simulink library "module_switch"  (R2013b)
settings: Solver=ode45  StartTime=0.0  StopTime=10.0  RelTol=1e-3
values from neighbouring files (symbols this model uses):
  D = (Vref - Vs) / Vref    (= 0.6)    [array_init.m]
  modes = 4    [array_init.m]
  T = 4e-6    (= 4e-06)    [array_init.m]
  Tstartup = 3e-3    (= 0.003)    [array_init.m]
libraries: fl_lib x6, nesl_utility x3, dspmtrx3 x1, elec_lib x1
settings Model: Creator=Taylor  LastModifiedBy=Luan Nguyen

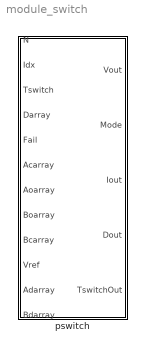
== system module_switch ==
  pswitch : Subsystem

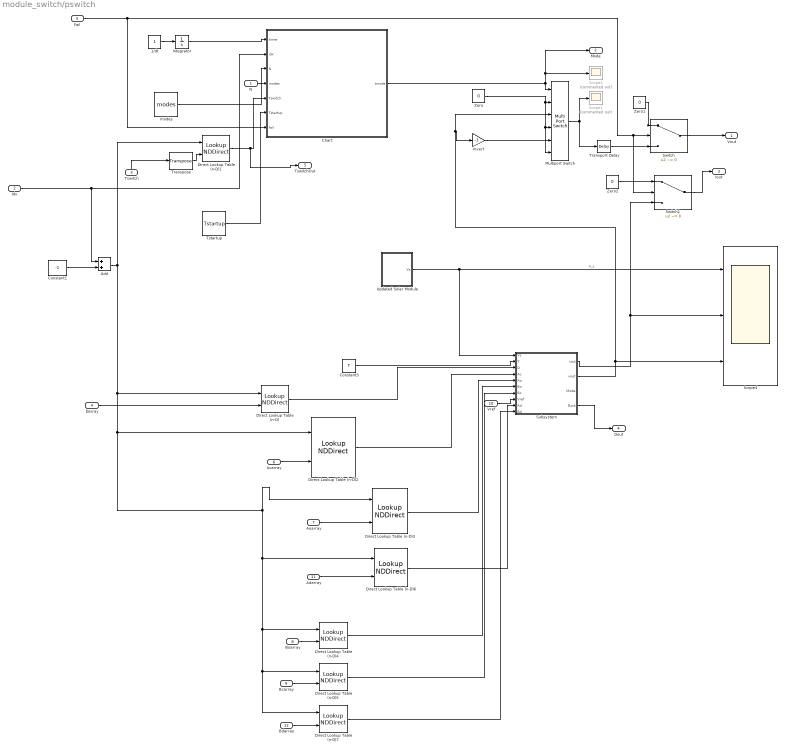
== system module_switch/pswitch ==
  N : Inport
  Idx : Inport  Port=2
  Tswitch : Inport  Port=3
  Darray : Inport  Port=4
  Fail : Inport  Port=5
  Acarray : Inport  Port=6
  Aoarray : Inport  Port=7
  Boarray : Inport  Port=8
  Bcarray : Inport  Port=9
  Vref : Inport  Port=10
  Adarray : Inport  Port=11
  Bdarray : Inport  Port=12
  1/dt : Constant
  Add : Sum
  Chart : Stateflow chart  TreatAsAtomicUnit=on
  Constant1 : Constant  Value=-1
  Constant3 : Constant  Value=T
  Direct Lookup Table (n-D) : LookupNDDirect  NumberOfTableDimensions=1  TableIsInput=on  Table=D
  Direct Lookup Table (n-D){1,4..5,7} (4 alike) : LookupNDDirect  InputsSelectThisObjectFromTable=Column  TableIsInput=on  Table=D
  Direct Lookup Table (n-D)2 : LookupNDDirect  NumberOfTableDimensions=3  InputsSelectThisObjectFromTable=2-D Matrix  TableIsInput=on  Table=D
  Direct Lookup Table (n-D)3 : LookupNDDirect  NumberOfTableDimensions=3  InputsSelectThisObjectFromTable=2-D Matrix  TableIsInput=on  Table=D
  Direct Lookup Table (n-D)6 : LookupNDDirect  NumberOfTableDimensions=3  InputsSelectThisObjectFromTable=2-D Matrix  TableIsInput=on
  Integrator : Integrator
  Invert : Gain  Gain=-1
  Multiport Switch : MultiPortSwitch  Inputs=4  DataPortForDefault=Additional data port  DiagnosticForDefault=None
  Scope1 : Scope  Commented=on
      settings: TimeRange=0.1  YMin=-2.1  YMax=0
  Scope2 : Scope  Commented=on
      settings: TimeRange=0.1  YMin=3  YMax=3  SaveName=ScopeData2
  Scope4 : Scope  NumInputPorts=3
      settings: TimeRange=0.005  YMin=17.75~2.5~14.2  YMax=22.75~14~15.7  SaveName=ScopeData4
  Subsystem : Subsystem
  Switch : Switch  Criteria=u2 ~= 0  Threshold=1
  Switch1 : Switch  Criteria=u2 ~= 0  Threshold=1
  Transport Delay : TransportDelay  DelayTime=1e-4
  Transpose : dspmtrx3/Transpose  Hermitian=off  overflowFlag=off
  Tstartup : Constant  Value=Tstartup
  Updated Solar Module : Subsystem
  Zero : Constant  Value=0
  Zero1 : Constant  Value=0
  Zero2 : Constant  Value=0
  modes : Constant  Value=modes
  Vout : Outport
  Mode : Outport  Port=2
  Iout : Outport  Port=3
  Dout : Outport  Port=4
  TswitchOut : Outport  Port=5
  wires:
  Invert/1 -> Multiport Switch/5
  Chart/1(tmode) -> Multiport Switch/1, Mode/1, Scope2/1
  Zero/1 -> Multiport Switch/6, Multiport Switch/4, Multiport Switch/2
  Multiport Switch/1 -> Transport Delay/1, Scope1/1
  N/1 -> Chart/3(N)
  modes/1 -> Chart/4(modes)
  Integrator/1 -> Chart/1(timer)
  1/dt/1 -> Integrator/1
  Idx/1 -> Chart/2(idx), Add/1
  Darray/1 -> Direct Lookup Table (n-D)/2
  Add/1 -> Direct Lookup Table (n-D)/1, Direct Lookup Table (n-D)2/1, Direct Lookup Table (n-D)3/1, Direct Lookup Table (n-D)6/1, Direct Lookup Table (n-D)7/1, Direct Lookup Table (n-D)5/1, Direct Lookup Table (n-D)4/1, Direct Lookup Table (n-D)1/1
  Constant1/1 -> Add/2
  Tswitch/1 -> Transpose/1
  Direct Lookup Table (n-D)1/1 -> TswitchOut/1, Chart/5(Tswitch)
  Transpose/1 -> Direct Lookup Table (n-D)1/2
  Fail/1 -> Chart/7(fail), Switch1/2, Switch/2
  Switch/1 -> Vout/1
  Zero1/1 -> Switch/1
  Zero2/1 -> Switch1/1
  Switch1/1 -> Iout/1
  Acarray/1 -> Direct Lookup Table (n-D)2/2
  Aoarray/1 -> Direct Lookup Table (n-D)3/2
  Boarray/1 -> Direct Lookup Table (n-D)4/2
  Bcarray/1 -> Direct Lookup Table (n-D)5/2
  Tstartup/1 -> Chart/6(Tstartup)
  Subsystem/1(iout) -> Switch1/3, Scope4/2
  Subsystem/2(vout) -> Multiport Switch/3, Invert/1, Scope4/3
  Constant3/1 -> Subsystem/2(T)
  Direct Lookup Table (n-D)/1 -> Subsystem/3(D)
  Direct Lookup Table (n-D)2/1 -> Subsystem/4(Ac)
  Direct Lookup Table (n-D)3/1 -> Subsystem/5(Ao)
  Direct Lookup Table (n-D)4/1 -> Subsystem/6(Bo)
  Direct Lookup Table (n-D)5/1 -> Subsystem/7(Bc)
  Vref/1 -> Subsystem/8(Vref)
  Subsystem/4(Dout) -> Dout/1
  Updated Solar Module/1(Vs) -> Subsystem/1(Vs), Scope4/1  "V_s"
  Direct Lookup Table (n-D)6/1 -> Subsystem/9(Ad)
  Adarray/1 -> Direct Lookup Table (n-D)6/2
  Bdarray/1 -> Direct Lookup Table (n-D)7/2
  Direct Lookup Table (n-D)7/1 -> Subsystem/10(Bd)
  Transport Delay/1 -> Switch/3

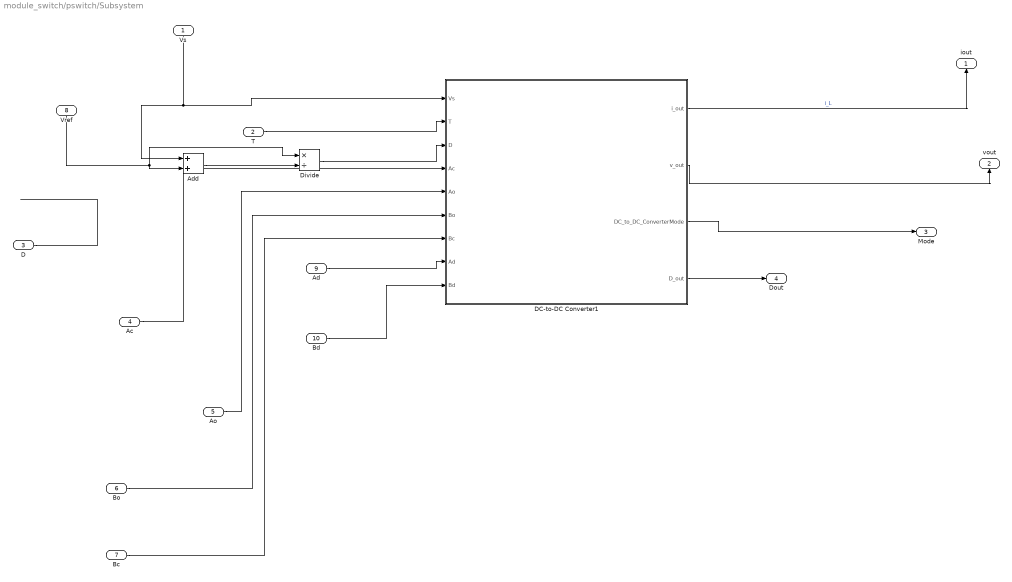
== system module_switch/pswitch/Subsystem ==
  Vs : Inport
  T : Inport  Port=2
  D : Inport  Port=3
  Ac : Inport  Port=4
  Ao : Inport  Port=5
  Bo : Inport  Port=6
  Bc : Inport  Port=7
  Vref : Inport  Port=8
  Ad : Inport  Port=9
  Bd : Inport  Port=10
  Add : Sum
  DC-to-DC Converter1 : Stateflow chart  TreatAsAtomicUnit=on
  Divide : Product  Inputs=*/
  iout : Outport
  vout : Outport  Port=2
  Mode : Outport  Port=3
  Dout : Outport  Port=4
  wires:
  DC-to-DC Converter1/3(DC_to_DC_ConverterMode) -> Mode/1
  Vs/1 -> DC-to-DC Converter1/1(Vs), Add/1
  T/1 -> DC-to-DC Converter1/2(T)
  D/1 -> ?
  Ac/1 -> DC-to-DC Converter1/4(Ac)
  Ao/1 -> DC-to-DC Converter1/5(Ao)
  DC-to-DC Converter1/1(i_out) -> iout/1  "i_L"
  Bc/1 -> DC-to-DC Converter1/7(Bc)
  DC-to-DC Converter1/2(v_out) -> vout/1
  Bo/1 -> DC-to-DC Converter1/6(Bo)
  Vref/1 -> Divide/1, Add/2
  Divide/1 -> DC-to-DC Converter1/3(D)
  Add/1 -> Divide/2
  DC-to-DC Converter1/4(D_out) -> Dout/1
  Ad/1 -> DC-to-DC Converter1/8(Ad)
  Bd/1 -> DC-to-DC Converter1/9(Bd)

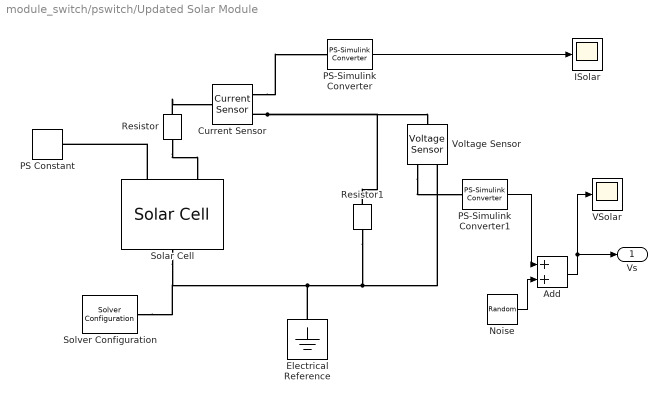
== system module_switch/pswitch/Updated Solar Module ==
  Add : Sum
  Current Sensor : fl_lib/Electrical/Electrical Sensors/Current Sensor  i1_Log=off  v1_Log=off  LocalVarNames=|i1|v1  LocalVarDescs=|i1|v1  LocalVarLogging=[0 0]
  Electrical Reference : fl_lib/Electrical/Electrical Elements/Electrical Reference  i_Log=off  LocalVarNames=|i  LocalVarDescs=|i  LocalVarLogging=0
  ISolar : Scope
  Noise : RandomNumber  Variance=0.2  SampleTime=1/T
  PS Constant : fl_lib/Physical Signals/Sources/PS Constant  constant=1000  LocalVarLogging=[]
  PS-Simulink Converter : nesl_utility/PS-Simulink Converter  PhysicalDomain=network_engine_domain  SubClassName=ps_output  LeftPortType=input  RightPortType=output  PseudoPeriodic=off  Frequencies=[]  Unit=1  AffineConversion=off
  PS-Simulink Converter1 : nesl_utility/PS-Simulink Converter  PhysicalDomain=network_engine_domain  SubClassName=ps_output  LeftPortType=input  RightPortType=output  PseudoPeriodic=off  Frequencies=[]  Unit=1  AffineConversion=off
  Resistor : fl_lib/Electrical/Electrical Elements/Resistor  R=1 Ohm  i_Log=off  v_Log=off  LocalVarNames=|i|v  LocalVarDescs=|i|v  LocalVarLogging=[0 0]
  Resistor1 : fl_lib/Electrical/Electrical Elements/Resistor  R=2 Ohm  i_Log=off  v_Log=off  LocalVarNames=|i|v  LocalVarDescs=|i|v  LocalVarLogging=[0 0]
  Solar Cell : elec_lib/Sources/Solar Cell  prm=1  Isc=6.13 A  Voc=21.9 V  Is=1e-6 A  Is2=0 A  Iph=7.34 A  Ir0=1000 W/m^2  ec=1.5  N2=2  Rs=0 Ohm  Rp=Inf Ohm  N_series=1  TIPH1=0 1/K  EG=1.11 eV  TXIS1=3  TXIS2=3  TRS1=0  TRP1=0  Tmeas=25 C  TFIXED=25 C  LocalVarLogging=[]  thermal_mass=100 J/K  initial_temperature=25 C
  Solver Configuration : nesl_utility/Solver Configuration  PhysicalDomain=network_engine_domain  SubClassName=solver  LeftPortType=input  RightPortType=generic  Accelerate=off  Tones=[]  Harmonics=[]  SimulateNoise=off  Profile=off  UseLocalSampling=off  EnableSwitchedLinearOptims=on  FrequencyDomain=off  UseCCode=off  RelTol=0.001  AbsTol=1e-06  MinStep=1e-09  ToWorkspace=off  DoDC=off  ResidualTolerance=1e-09  UseLocalSolver=off  LocalSolverChoice=NE_BACKWARD_EULER_ADVANCER  LocalSolverSampleTime=0.001  DoFixedCost=off  MaxNonlinIter=3  MaxModeIter=2  LinearAlgebra=Sparse  DelaysMemoryBudget=1024
  VSolar : Scope
  Voltage Sensor : fl_lib/Electrical/Electrical Sensors/Voltage Sensor  i1_Log=off  v1_Log=off  LocalVarNames=|i1|v1  LocalVarDescs=|i1|v1  LocalVarLogging=[0 0]
  Vs : Outport
  wires:
  PS-Simulink Converter/1 -> ISolar/1
  Noise/1 -> Add/2
  PS-Simulink Converter1/1 -> Add/1
  Add/1 -> Vs/1, VSolar/1
  connections:
  Solar Cell/LConn1 -- PS Constant/RConn1
  Current Sensor/RConn2 -- Resistor1/LConn1 -- Voltage Sensor/LConn1
  Resistor/LConn1 -- Current Sensor/LConn1
  Voltage Sensor/RConn1 -- PS-Simulink Converter1/LConn1
  Electrical Reference/LConn1 -- Solar Cell/RConn1 -- Solver Configuration/RConn1 -- Resistor1/RConn1 -- Voltage Sensor/RConn2
  Current Sensor/RConn1 -- PS-Simulink Converter/LConn1
  Resistor/RConn1 -- Solar Cell/LConn2

== stateflow chart module_switch/pswitch/Chart ==
  settings: updateMethod=CONTINUOUS
  state Negative
    du:
    clock_dot = 1;
  state Startup
  state Zero
    du:
    clock_dot = 1;
  state Positive
    du:
    clock_dot = 1;
  Negative -> Zero : [fail || (tmode == 4 && clock >= (Tswitch[0]+Tswitch[1]+Tswitch[2]+Tswitch[3]))]
      | {tmode=5;}
  Zero -> Negative [order 2] : [!fail && tmode == 3 && clock >= (Tswitch[0]+Tswitch[1]+Tswitch[2])]
      | {tmode = 4;}
  (default) -> Startup : {tmode=0; clock = 0;}
  Startup -> Zero : [tmode == 0 && after(Tstartup,sec)]
      | {tmode=1; clock = 0;}
  Zero -> Positive [order 3] : [!fail && (tmode == 1) && clock >= (Tswitch[0])]
      | {tmode=2; }
  Zero -> Positive [order 1] : [!fail && (tmode == 5) && clock >= (Tswitch[0]+Tswitch[1]+Tswitch[2]+Tswitch[3]+Tswitch[4])]
      | {tmode=2;  clock = Tswitch[0];}
  Positive -> Zero : [fail || (tmode == 2 && clock >= (Tswitch[0]+Tswitch[1]))]
      | {tmode=3;}
  data: timer input; idx input [0..N]; tmode output; N input [1..]; modes input [0..4]; Tswitch input [0..]; Tstartup input [0..]; clock local double; fail input
  data clock settings: updateMethod=SF_CONTINUOUS_TIME_DATA

== stateflow chart module_switch/pswitch/Subsystem/DC-to-DC Converter1 ==
  settings: updateMethod=CONTINUOUS
  state Discontinuous
    du:
    i_dot = Ad[0][0]*i+Ad[0][1]*v+Bd[0]*Vs;
    v_dot = Ad[1][0]*i+Ad[1][1]*v+Bd[1]*Vs;
    t_dot = 1;
    i_out = i;
    v_out = v;
    D_out=D;
  state Charging
    du:
    i_dot = Ac[0][0]*i+Ac[0][1]*v+Bc[0]*Vs;
    v_dot = Ac[1][0]*i+Ac[1][1]*v+Bc[1]*Vs;
    t_dot = 1;
    i_out = i;
    v_out = v;
    D_out=D;
  state Discharging
    du:
    i_dot = Ao[0][0]*i+Ao[0][1]*v+Bo[0]*Vs;
    v_dot = Ao[1][0]*i+Ao[1][1]*v+Bo[1]*Vs;
    t_dot = 1;
    i_out = i;
    v_out = v;
    D_out=D;
  Discharging -> Discontinuous [order 2] : [i <= 0]
  Discontinuous -> Charging : [t>= (1-D)*T]
      | {t= 0;}
  Charging -> Discharging : [t>= D*T]
      | {t= 0;}
  Discharging -> Charging [order 1] : [t>= (1-D)*T]
      | {t= 0;}
  (default) -> Charging : {i = 0;
      | v = 0;}
  data: t local double; i_out output double; v_out output double; i local double; Vs input double =120; T input double; D input double [0..1]; v local double; DC_to_DC_ConverterMode output Enum: DC_to_DC_ConverterModeType; Ac input double size=2,2; Ao input double size=2,2; Bo input double size=2,1; Bc input double size=2,1; D_out output double [0..1]; Ad input double size=2,2; Bd input double size=2,1
  data t settings: updateMethod=SF_CONTINUOUS_TIME_DATA
  data i settings: updateMethod=SF_CONTINUOUS_TIME_DATA
  data v settings: updateMethod=SF_CONTINUOUS_TIME_DATA
